simulink model "PID_container_model_Input_Params"  (R2016b)
settings: Solver=FixedStepDiscrete  StartTime=0.0  StopTime=7200  FixedStep=0.01  MaxStep=0.001  RelTol=1e-4  EnableMultiTasking=on
StartFcn:
  | CONSTANTS
values from neighbouring files (symbols this model uses):
  C = 1000    [CONSTANTS.m]
  Cc = 9100    [CONSTANTS.m]
  Ccov = 0.6    [CONSTANTS.m]
  Ch = 9100    [CONSTANTS.m]
  CK = 2    [CONSTANTS.m]
  Cp = 718    [CONSTANTS.m]
  H = 1000    [CONSTANTS.m]
  H_const = 0.0    (= 0)    [CONSTANTS.m]
  Hcov = 0.7    [CONSTANTS.m]
  HK = 5    [CONSTANTS.m]
  HTC = 0.5    [CONSTANTS.m]
  kd = 0    [CONSTANTS.m]
  ki = 0.01    [CONSTANTS.m]
  kp = 5    [CONSTANTS.m]
  mc = 0.113/2.45    (= 0.0461224489796)    [CONSTANTS.m]
  mh = 0.293/2    (= 0.1465)    [CONSTANTS.m]
  Qc = Cc * mc * T    (= 123396)    [CONSTANTS.m]    (also in heat_caps.m = 2*(To-Ti)/Rt; heat_caps2.m = (To-Ti)/Rt)
  Qh = Ch * mh * T    (= 391946.1)    [CONSTANTS.m]
  Qp = Cp*V*1.2754*T    (= 403.8401052)    [CONSTANTS.m]
  Rtc = 0.7    [CONSTANTS.m]
  Rth = 0.152    [CONSTANTS.m]
  Rtp = 6.25*0.8    (= 5)    [CONSTANTS.m]
  T = 294    [CONSTANTS.m]
  Target = 280    [CONSTANTS.m]
  V = .0015    (= 0.0015)    [CONSTANTS.m]
undefined symbols (not defined in the file or in its folder): DiscIntNeverNeededParam
libraries: simulink x1
settings Model: Creator=Evan  LastModifiedBy=Evan
settings DataIOCC: LimitDataPoints=on  SaveOutput=off  SaveTime=off
settings OptimizationCC: ExpressionDepthLimit=2147483647  LifeSpan=1
settings DebuggingCC: UnderspecifiedInitializationDetection=Classic  MergeDetectMultiDrivingBlocksExec=none  FcnCallInpInsideContextMsg=warning  AllowSymbolicDim=off  StateNameClashWarn=warning  SFUnexpectedBacktrackingDiag=warning  SFNoUnconditionalDefaultTransitionDiag=warning  SFExecutionAtInitializationDiag=none
settings GRTTargetCC: TargetLangStandard=C89/C90 (ANSI)  GeneratePreprocessorConditionals=Disable all  CombineOutputUpdateFcns=off  GRTInterface=on

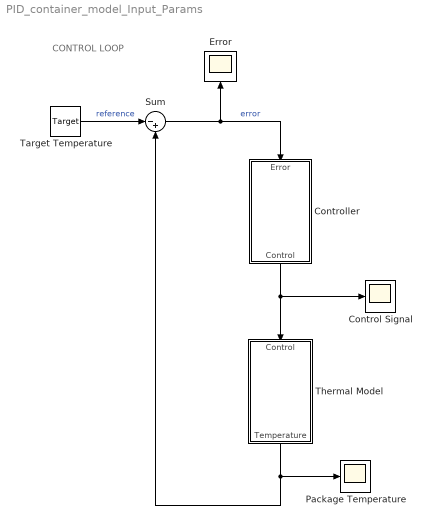
== system PID_container_model_Input_Params ==
  note: CONTROL
      | LOOP
  Control Signal : Scope
  Controller : Subsystem
  Error : Scope
  Package Temperature : Scope
  Sum : Sum  Inputs=|-+
  Target Temperature : Constant  Value=Target
  Thermal Model : Subsystem
  wires:
  Target Temperature/1 -> Sum/1  "reference"
  Controller/1(Control) -> Thermal Model/1(Control), Control Signal/1
  Sum/1 -> Error/1, Controller/1(Error)  "error"
  Thermal Model/1(Temperature) -> Sum/2, Package Temperature/1

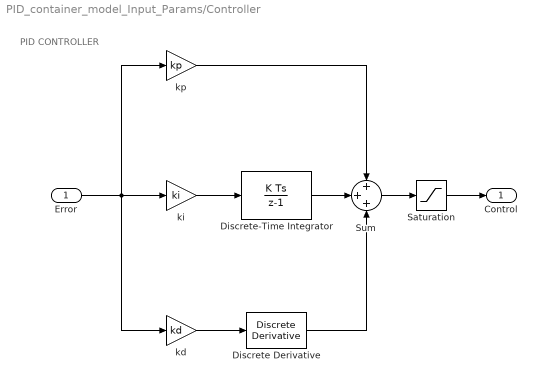
== system PID_container_model_Input_Params/Controller ==
  note: PID CONTROLLER
  Error : Inport
  Discrete Derivative : simulink/Discrete/Discrete Derivative  gainval=1.0  ICPrevScaledInput=0.0  OutMin=[]  OutMax=[]  OutDataType=fixdt(1, 16)  OutScaling=2^-10  DoSatur=off
  Discrete-Time Integrator : DiscreteIntegrator  InitialConditionSetting=State (most efficient)  SampleTime=-1  LimitOutput=on  UpperSaturationLimit=5  ICPrevOutput=DiscIntNeverNeededParam  ICPrevScaledInput=DiscIntNeverNeededParam
  Saturation : Saturate  UpperLimit=5  LowerLimit=0
  Sum : Sum  Inputs=+++
  kd : Gain  Gain=kd
  ki : Gain  Gain=ki
  kp : Gain  Gain=kp
  Control : Outport
  wires:
  Saturation/1 -> Control/1
  Error/1 -> kp/1, kd/1, ki/1
  ki/1 -> Discrete-Time Integrator/1
  kd/1 -> Discrete Derivative/1
  Sum/1 -> Saturation/1
  kp/1 -> Sum/1
  Discrete-Time Integrator/1 -> Sum/2
  Discrete Derivative/1 -> Sum/3

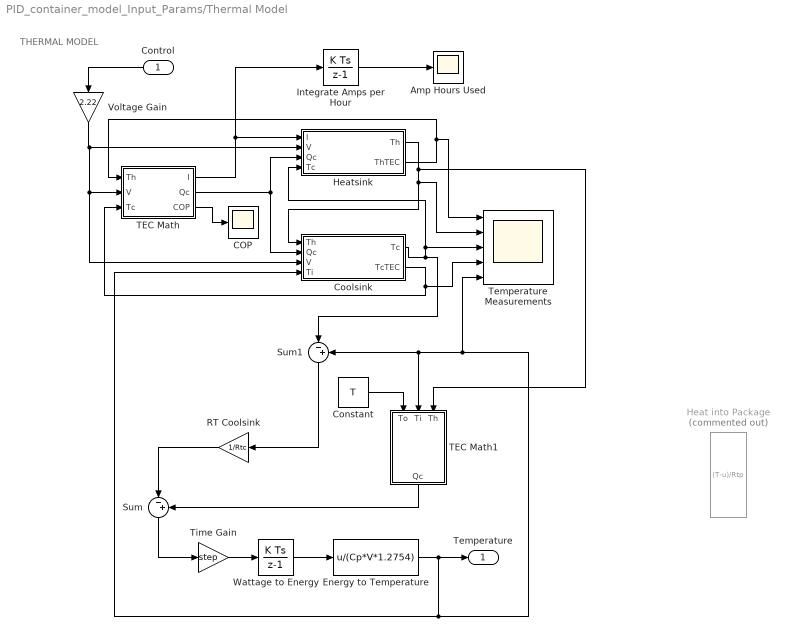
== system PID_container_model_Input_Params/Thermal Model ==
  note: THERMAL
      | MODEL
  Control : Inport
  Amp Hours Used : Scope
  COP : Scope
  Constant : Constant  Value=T
  Coolsink : Subsystem
  Energy to Temperature : Fcn  Expr=u/(Cp*V*1.2754)
  Heat into Package : Fcn  Commented=on  Expr=(T-u)/Rtp
  Heatsink : Subsystem
  Integrate Amps per Hour : DiscreteIntegrator  gainval=1/(3600)*step  InitialConditionSetting=State (most efficient)  SampleTime=-1  ICPrevOutput=DiscIntNeverNeededParam  ICPrevScaledInput=DiscIntNeverNeededParam
  "RT Coolsink " : Gain  Gain=1/Rtc
  Sum : Sum  Inputs=|-+
  Sum1 : Sum  Inputs=|-+
  TEC Math : MATLAB Function  TreatAsAtomicUnit=on
  TEC Math1 : MATLAB Function  TreatAsAtomicUnit=on
  Temperature Measurements : Scope  NumInputPorts=5
  Time Gain : Gain  Gain=step
  Voltage Gain : Gain  Gain=2.22
  Wattage to Energy : DiscreteIntegrator  InitialCondition=Qp  InitialConditionSetting=State (most efficient)  SampleTime=-1  ICPrevOutput=DiscIntNeverNeededParam  ICPrevScaledInput=DiscIntNeverNeededParam
  Temperature : Outport
  wires:
  Control/1 -> Voltage Gain/1
  Voltage Gain/1 -> TEC Math/2(V), Coolsink/3(V), Heatsink/2(V)
  TEC Math/2(Qc) -> Heatsink/3(Qc), Coolsink/2(Qc)
  TEC Math/1(I) -> Integrate Amps per Hour/1, Heatsink/1(I)
  TEC Math1/1(Qc) -> Sum/2
  Sum/1 -> Time Gain/1
  Time Gain/1 -> Wattage to Energy/1
  Wattage to Energy/1 -> Energy to Temperature/1
  Coolsink/1(Tc) -> Heatsink/4(Tc), Temperature Measurements/3, Sum1/1
  "RT Coolsink "/1 -> Sum/1
  Energy to Temperature/1 -> Temperature/1, Temperature Measurements/5, Sum1/2, TEC Math1/2(Ti), Coolsink/4(Ti)
  TEC Math/3(COP) -> COP/1
  Integrate Amps per Hour/1 -> Amp Hours Used/1
  Sum1/1 -> "RT Coolsink "/1
  Heatsink/2(ThTEC) -> Temperature Measurements/1, TEC Math/1(Th)
  Coolsink/2(TcTEC) -> Temperature Measurements/4, TEC Math/3(Tc)
  Heatsink/1(Th) -> TEC Math1/3(Th), Temperature Measurements/2, Coolsink/1(Th)
  Constant/1 -> TEC Math1/1(To)

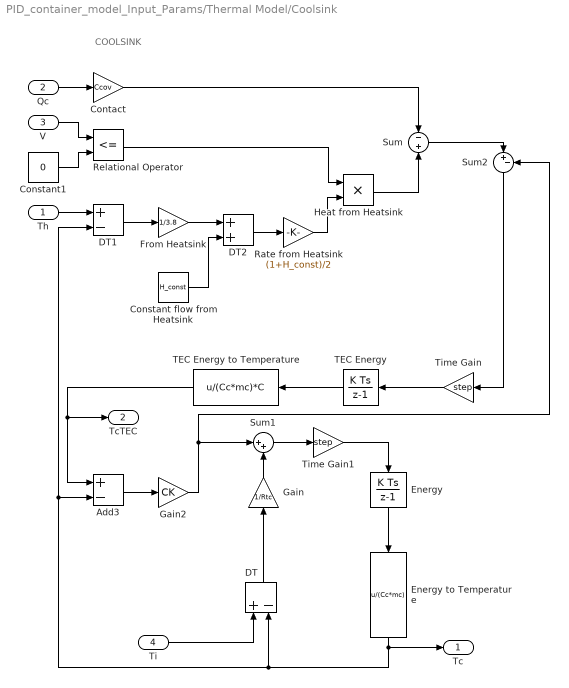
== system PID_container_model_Input_Params/Thermal Model/Coolsink ==
  note: COOLSINK
  Th : Inport
  Qc : Inport  Port=2
  V : Inport  Port=3
  Ti : Inport  Port=4
  Add3 : Sum  Inputs=+-
  Constant flow from Heatsink : Constant  Value=H_const
  Constant1 : Constant  Value=0
  Contact : Gain  Gain=Ccov
  DT : Sum  Inputs=+-
  DT1 : Sum  Inputs=+-
  DT2 : Sum
  Energy : DiscreteIntegrator  InitialCondition=Qc  InitialConditionSetting=State (most efficient)  SampleTime=-1  ICPrevOutput=DiscIntNeverNeededParam  ICPrevScaledInput=DiscIntNeverNeededParam
  Energy to Temperature : Fcn  Expr=u/(Cc*mc)
  From Heatsink : Gain  Gain=1/3.8
  Gain : Gain  Gain=1/Rtc
  Gain2 : Gain  Gain=CK
  Heat from Heatsink : Product
  Rate from Heatsink : Gain  Gain=(1+H_const)/2
  Relational Operator : RelationalOperator  Operator=<=  OutDataTypeStr=boolean  RndMeth=Simplest
  Sum : Sum  Inputs=-+
  Sum1 : Sum  Inputs=|++
  Sum2 : Sum  Inputs=|+-
  TEC Energy : DiscreteIntegrator  InitialCondition=Qc/C  InitialConditionSetting=State (most efficient)  SampleTime=-1  ICPrevOutput=DiscIntNeverNeededParam  ICPrevScaledInput=DiscIntNeverNeededParam
  TEC Energy to Temperature : Fcn  Expr=u/(Cc*mc)*C
  Time Gain : Gain  Gain=step
  Time Gain1 : Gain  Gain=step
  Tc : Outport
  TcTEC : Outport  Port=2
  wires:
  Energy/1 -> Energy to Temperature/1
  Qc/1 -> Contact/1
  Contact/1 -> Sum/1
  DT/1 -> Gain/1
  Gain/1 -> Sum1/2
  Th/1 -> DT1/1
  DT1/1 -> From Heatsink/1
  Constant1/1 -> Relational Operator/2
  Heat from Heatsink/1 -> Sum/2
  V/1 -> Relational Operator/1
  Relational Operator/1 -> Heat from Heatsink/1
  DT2/1 -> Rate from Heatsink/1
  From Heatsink/1 -> DT2/1
  Rate from Heatsink/1 -> Heat from Heatsink/2
  Constant flow from Heatsink/1 -> DT2/2
  TEC Energy/1 -> TEC Energy to Temperature/1
  Ti/1 -> DT/1
  TEC Energy to Temperature/1 -> Add3/1, TcTEC/1
  Energy to Temperature/1 -> Tc/1, Add3/2, DT1/2, DT/2
  Sum2/1 -> Time Gain/1
  Gain2/1 -> Sum1/1, Sum2/2
  Add3/1 -> Gain2/1
  Sum/1 -> Sum2/1
  Sum1/1 -> Time Gain1/1
  Time Gain/1 -> TEC Energy/1
  Time Gain1/1 -> Energy/1

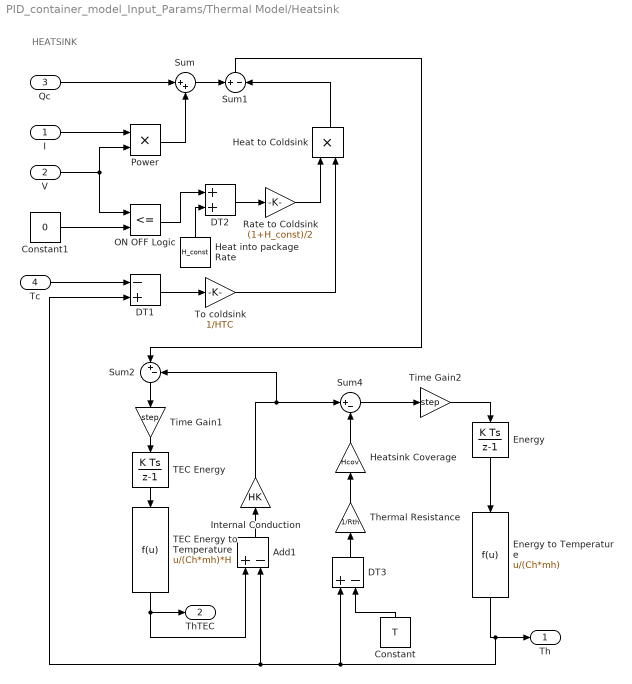
== system PID_container_model_Input_Params/Thermal Model/Heatsink ==
  note: HEATSINK
  I : Inport
  V : Inport  Port=2
  Qc : Inport  Port=3
  Tc : Inport  Port=4
  Add1 : Sum  Inputs=+-
  Constant : Constant  Value=T
  Constant1 : Constant  Value=0
  DT1 : Sum  Inputs=-+
  DT2 : Sum
  DT3 : Sum  Inputs=+-
  Energy : DiscreteIntegrator  InitialCondition=Qh  InitialConditionSetting=State (most efficient)  SampleTime=-1  ICPrevOutput=DiscIntNeverNeededParam  ICPrevScaledInput=DiscIntNeverNeededParam
  Energy to Temperature : Fcn  Expr=u/(Ch*mh)
  Heat into package Rate : Constant  Value=H_const
  Heat to Coldsink : Product
  Heatsink Coverage : Gain  Gain=Hcov
  Internal Conduction : Gain  Gain=HK
  ON OFF Logic : RelationalOperator  Operator=<=  OutDataTypeStr=boolean  RndMeth=Simplest
  Power : Product
  Rate to Coldsink : Gain  Gain=(1+H_const)/2
  Sum : Sum  Inputs=|++
  Sum1 : Sum  Inputs=+-
  Sum2 : Sum  Inputs=|+-
  Sum4 : Sum  Inputs=|+-
  TEC Energy : DiscreteIntegrator  InitialCondition=Qh/H  InitialConditionSetting=State (most efficient)  SampleTime=-1  ICPrevOutput=DiscIntNeverNeededParam  ICPrevScaledInput=DiscIntNeverNeededParam
  TEC Energy to Temperature : Fcn  Expr=u/(Ch*mh)*H
  Thermal Resistance : Gain  Gain=1/Rth
  Time Gain1 : Gain  Gain=step
  Time Gain2 : Gain  Gain=step
  To coldsink : Gain  Gain=1/HTC
  Th : Outport
  ThTEC : Outport  Port=2
  wires:
  Qc/1 -> Sum/1
  Power/1 -> Sum/2
  V/1 -> ON OFF Logic/1, Power/2
  Energy/1 -> Energy to Temperature/1
  I/1 -> Power/1
  DT1/1 -> To coldsink/1
  Tc/1 -> DT1/1
  Sum/1 -> Sum1/1
  Constant1/1 -> ON OFF Logic/2
  To coldsink/1 -> Heat to Coldsink/2
  Heat to Coldsink/1 -> Sum1/2
  ON OFF Logic/1 -> DT2/1
  Heat into package Rate/1 -> DT2/2
  DT2/1 -> Rate to Coldsink/1
  Rate to Coldsink/1 -> Heat to Coldsink/1
  TEC Energy/1 -> TEC Energy to Temperature/1
  TEC Energy to Temperature/1 -> Add1/1, ThTEC/1
  Add1/1 -> Internal Conduction/1
  Internal Conduction/1 -> Sum4/1, Sum2/2
  Sum1/1 -> Sum2/1
  Heatsink Coverage/1 -> Sum4/2
  DT3/1 -> Thermal Resistance/1
  Energy to Temperature/1 -> DT3/1, DT1/2, Add1/2, Th/1
  Constant/1 -> DT3/2
  Thermal Resistance/1 -> Heatsink Coverage/1
  Sum4/1 -> Time Gain2/1
  Sum2/1 -> Time Gain1/1
  Time Gain1/1 -> TEC Energy/1
  Time Gain2/1 -> Energy/1

== matlab function PID_container_model_Input_Params/Thermal Model/TEC Math1 ==
  data: To input; Qc output; Ti input; Th input
function Qc  = fcn(To,Ti,Th)
%{
Heat Transfer Program
Runs heat transfer analysis on a cylindrical package with internal
insulation.

Evan Bosia
%}

%Material Thickness
ti = 1 * 0.0254;
ts = 0.625/2 * 0.0254;

rs = 4 * 0.0254; %inner radius of structural pipe

h = 5.5 * 0.0254; % height of the structural container

v_air = 0;

%Material conduction coeff
ki = 0.05; %insulating material ~ Neoprene 0.05
ks = 0.19; %structural material ~ ABS = 0.10
           %PVC = 0.19

%Heat transfer analysis
Qw = heat_cylinder(rs, ti, ts, v_air, ki, ks, To, Ti, h);
Qc1 = 0.5 * heat_caps(rs, ti, ts, v_air, ki, 0.1, To, Ti);
Qc2 = heat_caps2(rs, ti, 0.004, ki, 0.1, Th, Ti);

Qc = Qw + Qc1 + Qc2;

Qc = Qc;

end

== matlab function PID_container_model_Input_Params/Thermal Model/TEC Math ==
  data: Th input; I output; V input; Tc input; Qc output; COP output
function [I, Qc, COP] = fcn(Th, V, Tc)
%{
TEC Math
This function runs TEC math to get the current draw, the heat transfer
rate, and the coefficient of performance.

Parameters: temperature hot side, voltage, temperature cold side

Returns: current, heat transfer rate, coefficient of performance

Evan Bosia
%}

n = 127;    %number of TEC couples in new TEC
Inew = 4.8; %Imax of new TEC

%Constants for TEC with 71 couples and Imax of 6 amps
s1 = 1.33450 * 10^-2; 
s2 = -5.37574 * 10^-5; 
s3 = 7.42731 * 10^-7;
s4 = -1.27141 * 10^-9;

r1 = 2.08317; 
r2 = -1.98763 * 10^-2; 
r3 = 8.53832 * 10^-5; 
r4 = -9.03143 * 10^-8;

k1 = 4.76218 * 10^-1;
k2 = -3.89821 * 10^-6;
k3 = -8.64864 * 10^-6;
k4 = 2.20869 * 10^-8;

%Temperature difference between hot and cold side
DT = (Th-Tc);

%Equations dependent on temperature difference
if(DT == 0)
    T = Th;
    Sm = s1 + s2*T + s3*T^2 + s4*T^3;
    Rm = r1 + r2*T + r3*T^2 + r4*T^3;
    Km = k1 + k2*T + k3*T^2 + k4*T^3;
else
    Smh = s1*Th + (s2*Th^2)/2 + (s3*Th^3)/3 + (s4*Th^4)/4;
    Smc = s1*Tc + (s2*Tc^2)/2 + (s3*Tc^3)/3 + (s4*Tc^4)/4;
    Sm = (Smh - Smc)/DT;

    Rmh = r1*Th + (r2*Th^2)/2 + (r3*Th^3)/3 + (r4*Th^4)/4;
    Rmc = r1*Tc + (r2*Tc^2)/2 + (r3*Tc^3)/3 + (r4*Tc^4)/4;
    Rm = (Rmh - Rmc)/DT;

    Kmh = k1*Th + (k2*Th^2)/2 + (k3*Th^3)/3 + (k4*Th^4)/4;
    Kmc = k1*Tc + (k2*Tc^2)/2 + (k3*Tc^3)/3 + (k4*Tc^4)/4;
    Km = (Kmh - Kmc)/DT;
end

%Convert to new TEC
Sm = Sm * (n/71);
Rm = Rm * (n/71) * (6/Inew);
Km = Km * (n/71) * (Inew/6);

%Current
I = (V - (Sm * DT))/Rm;

%Heat transfer rate
Qc = ((Sm * Tc * I) - (0.5 * I^2 * Rm) - (Km * DT));

%Power
P = I*V;

%If the current is negative, set power to a high value
if(P <= 0)
   P = 1000000; 
end

%If the TEC is unpowered, set Qc to the -temperature differential * Rt, I
%to 0 and COP to 0
if(V <= 0)
    Qc = -DT/1.6;
    I = 0;
    COP = 0;
else
    COP = Qc / P;
end

end
